simulink model "Segway"  (R2018b)
settings: Solver=VariableStepAuto  StartTime=0.0  StopTime=10.0  RelTol=1e-3
values from neighbouring files (symbols this model uses):
  a_1 = 1    [segway.m]
  beta0 = 2    [segway.m]
  l_p = 1    [segway.m]
  m_p = 1    [segway.m]
  m_w = 1.5    [segway.m]
  r = 0.2    [segway.m]
  theta0 = 0.6    [segway.m]
  theta_ref = 0.5    [segway.m]
undefined symbols (not defined in the file or in its folder): g, thetadot0
libraries: simulink x2
settings Model: Creator=Agurken  LastModifiedBy=Agurken
settings SolverCC: ZeroCrossAlgorithm=Adaptive
settings DebuggingCC: IgnoredZcDiagnostic=none

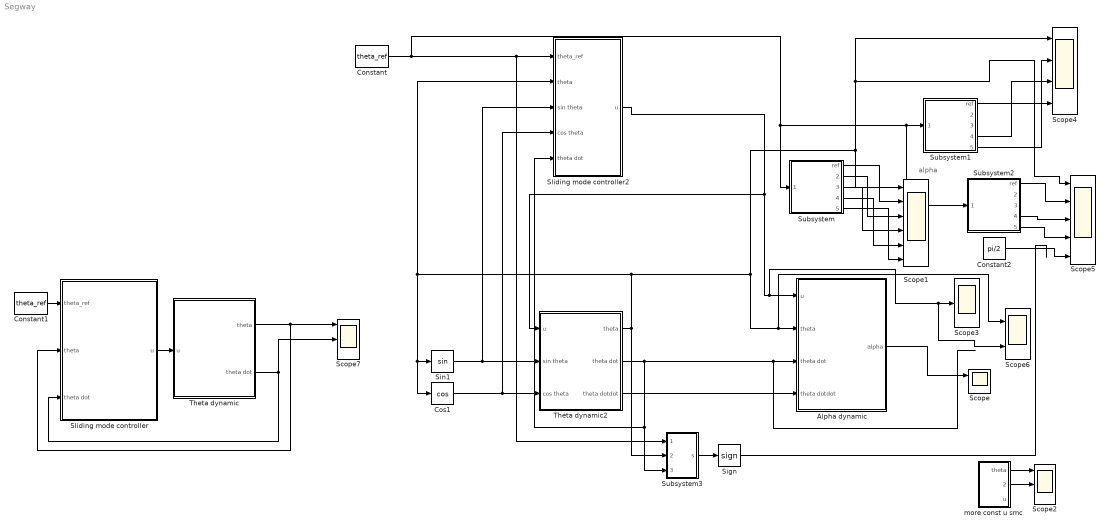
== system Segway ==
  note: alpha
  Alpha dynamic : Subsystem
  Constant : Constant  Value=theta_ref
  Constant1 : Constant  Value=theta_ref
  Constant2 : Constant  Value=pi/2
  Cos1 : Trigonometry  Operator=cos
  Scope : Scope  NumInputPorts=2
  Scope1 : Scope  NumInputPorts=6
  Scope2 : Scope  NumInputPorts=3
  Scope3 : Scope
  Scope4 : Scope  NumInputPorts=4
  Scope5 : Scope  NumInputPorts=5
  Scope6 : Scope  NumInputPorts=2
  Scope7 : Scope  NumInputPorts=3
  Sign : Signum
  Sin1 : Trigonometry
  Sliding mode controller : Subsystem
  Sliding mode controller2 : Subsystem
  Subsystem : Subsystem
  Subsystem1 : Subsystem
  Subsystem2 : Subsystem
  Subsystem3 : Subsystem
  Theta dynamic : Subsystem
  Theta dynamic2 : Subsystem
  more const u smc : Subsystem
  wires:
  Alpha dynamic/1(alpha) -> Scope/1
  Theta dynamic2/1("theta ") -> Subsystem3/2(theta), Sin1/1, Cos1/1, Sliding mode controller2/2(theta), Scope5/1, Scope4/1, Scope1/1, Scope6/1, Alpha dynamic/2(theta)
  Theta dynamic2/3("theta dotdot ") -> Alpha dynamic/4(theta dotdot)
  Cos1/1 -> Sliding mode controller2/4(cos theta), Theta dynamic2/3(cos theta)
  Sin1/1 -> Sliding mode controller2/3(sin theta), Theta dynamic2/2(sin theta)
  Sliding mode controller2/1(u) -> Scope6/2, Scope3/1, Alpha dynamic/1(u), Theta dynamic2/1(u)
  Constant/1 -> Subsystem3/1(theta_ref), Sliding mode controller2/1(theta_ref), Subsystem2/1(theta ref), Subsystem1/1(theta ref), Subsystem/1(theta ref)
  more const u smc/1(theta) -> Scope2/1
  more const u smc/2(theta ref) -> Scope2/2
  Subsystem/2(ref-eps) -> Scope1/3
  Subsystem/3(ref+epf) -> Scope1/4
  Subsystem/1(ref) -> Scope1/2
  Subsystem/5(ref+epf/a) -> Scope1/6
  Subsystem/4(ref-eps/a) -> Scope1/5
  Subsystem1/1(ref) -> Scope4/2
  Subsystem1/4(ref-eps/a) -> Scope4/3
  Subsystem1/5(ref+epf/a) -> Scope4/4
  Constant2/1 -> Scope5/5
  Subsystem2/4(ref-eps/a) -> Scope5/3
  Subsystem2/5(ref+epf/a) -> Scope5/4
  Subsystem2/1(ref) -> Scope5/2
  Subsystem3/1(s) -> Sign/1
  Sign/1 -> ?
  Sliding mode controller/1(u) -> Theta dynamic/1(u)
  Constant1/1 -> Sliding mode controller/1(theta_ref)
  Theta dynamic/1("theta ") -> Scope7/1, Sliding mode controller/2(theta)
  Theta dynamic/2("theta dot ") -> Scope7/2, Sliding mode controller/3(theta dot)
  Theta dynamic2/2("theta dot ") -> Subsystem3/3(theta dot), Sliding mode controller2/5(theta dot), Alpha dynamic/3(theta dot)

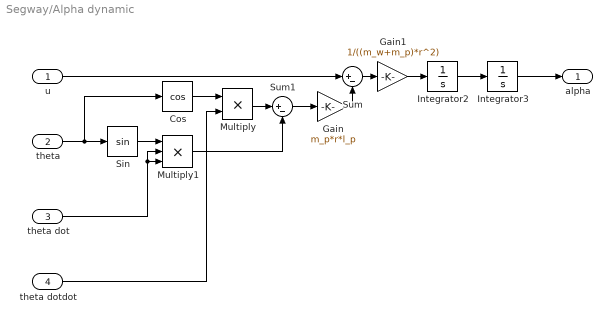
== system Segway/Alpha dynamic ==
  u : Inport
  theta : Inport  Port=2
  theta dot : Inport  Port=3
  theta dotdot : Inport  Port=4
  Cos : Trigonometry  Operator=cos
  Gain : Gain  Gain=m_p*r*l_p
  Gain1 : Gain  Gain=1/((m_w+m_p)*r^2)
  Integrator2 : Integrator
  Integrator3 : Integrator
  Multiply : Product
  Multiply1 : Product  Inputs=3
  Sin : Trigonometry
  Sum : Sum  Inputs=|+-
  Sum1 : Sum  Inputs=|+-
  alpha : Outport
  wires:
  Integrator2/1 -> Integrator3/1
  Multiply1/1 -> Sum1/2
  Multiply/1 -> Sum1/1
  Cos/1 -> Multiply/1
  Gain1/1 -> Integrator2/1
  Sin/1 -> Multiply1/1
  theta/1 -> Sin/1, Cos/1
  Sum1/1 -> Gain/1
  Sum/1 -> Gain1/1
  Gain/1 -> Sum/2
  u/1 -> Sum/1
  Integrator3/1 -> alpha/1
  theta dotdot/1 -> Multiply/2
  theta dot/1 -> Multiply1/3, Multiply1/2

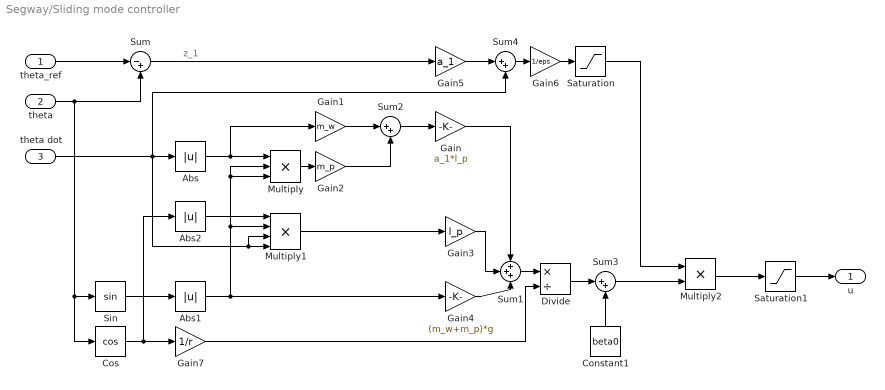
== system Segway/Sliding mode controller ==
  note: z_1
  theta_ref : Inport
  theta : Inport  Port=2
  theta dot : Inport  Port=3
  Abs : Abs
  Abs1 : Abs
  Abs2 : Abs
  Constant1 : Constant  Value=beta0
  Cos : Trigonometry  Operator=cos
  Divide : Product  Inputs=*/
  Gain : Gain  Gain=a_1*l_p
  Gain1 : Gain  Gain=m_w
  Gain2 : Gain  Gain=m_p
  Gain3 : Gain  Gain=l_p
  Gain4 : Gain  Gain=(m_w+m_p)*g
  Gain5 : Gain  Gain=a_1
  Gain6 : Gain  Gain=1/eps
  Gain7 : Gain  Gain=1/r
  Multiply : Product  Inputs=3
  Multiply1 : Product  Inputs=4
  Multiply2 : Product
  Saturation : Saturate  UpperLimit=1  LowerLimit=-1
  Saturation1 : Saturate  UpperLimit=1000  LowerLimit=-1000
  Sin : Trigonometry
  Sum : Sum  Inputs=|-+
  Sum1 : Sum  Inputs=3
  Sum2 : Sum  Inputs=|++
  Sum3 : Sum  Inputs=|++
  Sum4 : Sum  Inputs=|++
  u : Outport
  wires:
  Abs1/1 -> Multiply1/2, Multiply/3, Multiply/2, Gain4/1
  Sum1/1 -> Divide/1
  Sum2/1 -> Gain/1
  Sum3/1 -> Multiply2/2
  Gain3/1 -> Sum1/2
  theta dot/1 -> Multiply1/3, Multiply1/4, Abs/1, Sum4/2
  Gain6/1 -> Saturation/1
  Sum4/1 -> Gain6/1
  Multiply/1 -> Gain2/1
  Abs/1 -> Multiply/1, Gain1/1
  Saturation/1 -> Multiply2/1
  Gain2/1 -> Sum2/2
  Multiply2/1 -> Saturation1/1
  Multiply1/1 -> Gain3/1
  Gain5/1 -> Sum4/1
  Gain/1 -> Sum1/1
  Gain1/1 -> Sum2/1
  Gain4/1 -> Sum1/3
  Sin/1 -> Abs1/1
  Constant1/1 -> Sum3/2
  Cos/1 -> Gain7/1, Abs2/1
  theta/1 -> Cos/1, Sin/1, Sum/2
  theta_ref/1 -> Sum/1
  Gain7/1 -> Divide/2
  Divide/1 -> Sum3/1
  Saturation1/1 -> u/1
  Abs2/1 -> Multiply1/1
  Sum/1 -> Gain5/1

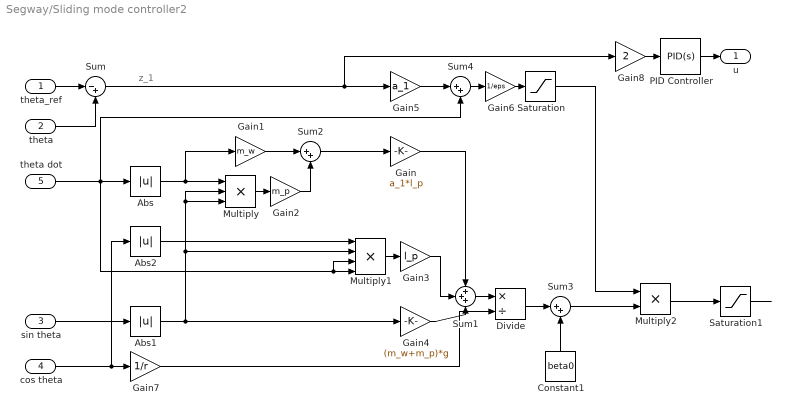
== system Segway/Sliding mode controller2 ==
  note: z_1
  theta_ref : Inport
  theta : Inport  Port=2
  sin theta : Inport  Port=3
  cos theta : Inport  Port=4
  theta dot : Inport  Port=5
  Abs : Abs
  Abs1 : Abs
  Abs2 : Abs
  Constant1 : Constant  Value=beta0
  Divide : Product  Inputs=*/
  Gain : Gain  Gain=a_1*l_p
  Gain1 : Gain  Gain=m_w
  Gain2 : Gain  Gain=m_p
  Gain3 : Gain  Gain=l_p
  Gain4 : Gain  Gain=(m_w+m_p)*g
  Gain5 : Gain  Gain=a_1
  Gain6 : Gain  Gain=1/eps
  Gain7 : Gain  Gain=1/r
  Gain8 : Gain  Gain=2
  Multiply : Product  Inputs=3
  Multiply1 : Product  Inputs=4
  Multiply2 : Product
  PID Controller : simulink/Continuous/PID Controller  Controller=PID  Form=Parallel  TimeDomain=Continuous-time  SampleTime=-1  IntegratorMethod=Forward Euler  FilterMethod=Forward Euler  ControllerParametersSource=internal  P=10  I=0  D=3  UseFilter=on  N=100  TunerSelectOption=Transfer Function Based (PID Tuner App)  InitialConditionSource=internal  InitialConditionForIntegrator=0  InitialConditionForFilter=0  DifferentiatorICPrevScaledInput=0  ExternalReset=none  TrackingMode=off  Kt=1  LimitOutput=off  UpperSaturationLimit=inf  LowerSaturationLimit=-inf  LinearizeAsGain=on  AntiWindupMode=none  Kb=1  POutMin=[]  POutMax=[]  IOutMin=[]  IOutMax=[]  DOutMin=[]  DOutMax=[]  NOutMin=[]  NOutMax=[]  SumOutMin=[]  SumOutMax=[]  SaturationOutMin=[]  SaturationOutMax=[]  PParamMin=[]  PParamMax=[]  IParamMin=[]  IParamMax=[]  DParamMin=[]  DParamMax=[]  NParamMin=[]  NParamMax=[]  KbParamMin=[]  KbParamMax=[]  KtParamMin=[]  KtParamMax=[]  KbOutMin=[]  KbOutMax=[]  KtOutMin=[]  KtOutMax=[]  IntegratorOutMin=[]  IntegratorOutMax=[]  FilterOutMin=[]  FilterOutMax=[]  SumI1OutMin=[]  SumI1OutMax=[]  SumI2OutMin=[]  SumI2OutMax=[]  SumI3OutMin=[]  SumI3OutMax=[]  SumI4OutMin=[]  SumI4OutMax=[]  SumDOutMin=[]  SumDOutMax=[]  DifferentiatorOutMin=[]  DifferentiatorOutMax=[]  FilterDiffOutCoefMin=[]  FilterDiffOutCoefMax=[]  ReciprocalOutMin=[]  ReciprocalOutMax=[]  SumDenOutMin=[]  SumDenOutMax=[]  SumNumOutMin=[]  SumNumOutMax=[]  DivideOutMin=[]  DivideOutMax=[]  IntegratorContinuousStateAttributes=''  IntegratorStateMustResolveToSignalObject=off  IntegratorRTWStateStorageClass=Auto  FilterContinuousStateAttributes=''  FilterStateMustResolveToSignalObject=off  FilterRTWStateStorageClass=Auto  ParallelPVariant=InternalParameters  IdealPVariant=Disabled  IVariant=InternalParameters  DVariant=InternalParameters  IntegratorVariant=Continuous  SatVariant=Disabled  AWVariant=Passthrough  PCopyVariant=Disabled  TRVariant=Disabled  FdbkBlocksVariant=Forward  IdealPFdbkVariant=Disabled  SatFdbkVariant=Disabled  DerivativeFilterVariant=ContFilter  NVariant=InternalParameters  NCopyVariant=Disabled  FilterICVariant=InternalICsFilter  IntegratorICVariant=InternalICs  ExternalResetVariant=Disabled  TRSumVariant=Passthrough  SumFdbkVariant=Disabled  SumVariant=Sum_PID
  Saturation : Saturate  UpperLimit=1  LowerLimit=-1
  Saturation1 : Saturate  UpperLimit=1000  LowerLimit=-1000
  Sum : Sum  Inputs=|-+
  Sum1 : Sum  Inputs=3
  Sum2 : Sum  Inputs=|++
  Sum3 : Sum  Inputs=|++
  Sum4 : Sum  Inputs=|++
  u : Outport
  wires:
  Abs1/1 -> Multiply1/2, Multiply/3, Multiply/2, Gain4/1
  Sum1/1 -> Divide/1
  Sum2/1 -> Gain/1
  Sum3/1 -> Multiply2/2
  Gain3/1 -> Sum1/2
  theta dot/1 -> Multiply1/4, Multiply1/3, Abs/1, Sum4/2
  Gain6/1 -> Saturation/1
  Sum4/1 -> Gain6/1
  Multiply/1 -> Gain2/1
  Abs/1 -> Multiply/1, Gain1/1
  Saturation/1 -> Multiply2/1
  Gain2/1 -> Sum2/2
  Multiply2/1 -> Saturation1/1
  Multiply1/1 -> Gain3/1
  Gain5/1 -> Sum4/1
  Gain/1 -> Sum1/1
  Gain1/1 -> Sum2/1
  Gain4/1 -> Sum1/3
  sin theta/1 -> Abs1/1
  Constant1/1 -> Sum3/2
  cos theta/1 -> Abs2/1, Gain7/1
  theta/1 -> Sum/2
  theta_ref/1 -> Sum/1
  Divide/1 -> Sum3/1
  Saturation1/1 -> ?
  Abs2/1 -> Multiply1/1
  PID Controller/1 -> u/1
  Sum/1 -> Gain8/1, Gain5/1
  Gain7/1 -> Divide/2
  Gain8/1 -> PID Controller/1

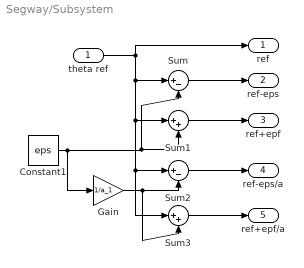
== system Segway/Subsystem ==
  theta ref : Inport
  Constant1 : Constant  Value=eps
  Gain : Gain  Gain=1/a_1
  Sum : Sum  Inputs=|+-
  Sum1 : Sum  Inputs=|++
  Sum2 : Sum  Inputs=|+-
  Sum3 : Sum  Inputs=|++
  ref : Outport
  ref-eps : Outport  Port=2
  ref+epf : Outport  Port=3
  ref-eps/a : Outport  Port=4
  ref+epf/a : Outport  Port=5
  wires:
  Sum1/1 -> ref+epf/1
  Constant1/1 -> Gain/1, Sum/2, Sum1/2
  Sum/1 -> ref-eps/1
  theta ref/1 -> ref/1, Sum/1, Sum1/1, Sum2/1, Sum3/1
  Gain/1 -> Sum3/2, Sum2/2
  Sum2/1 -> ref-eps/a/1
  Sum3/1 -> ref+epf/a/1

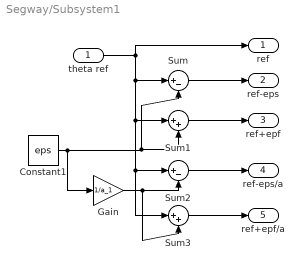
== system Segway/Subsystem1 ==
  theta ref : Inport
  Constant1 : Constant  Value=eps
  Gain : Gain  Gain=1/a_1
  Sum : Sum  Inputs=|+-
  Sum1 : Sum  Inputs=|++
  Sum2 : Sum  Inputs=|+-
  Sum3 : Sum  Inputs=|++
  ref : Outport
  ref-eps : Outport  Port=2
  ref+epf : Outport  Port=3
  ref-eps/a : Outport  Port=4
  ref+epf/a : Outport  Port=5
  wires:
  Sum1/1 -> ref+epf/1
  Constant1/1 -> Gain/1, Sum/2, Sum1/2
  Sum/1 -> ref-eps/1
  theta ref/1 -> ref/1, Sum/1, Sum1/1, Sum2/1, Sum3/1
  Gain/1 -> Sum3/2, Sum2/2
  Sum2/1 -> ref-eps/a/1
  Sum3/1 -> ref+epf/a/1

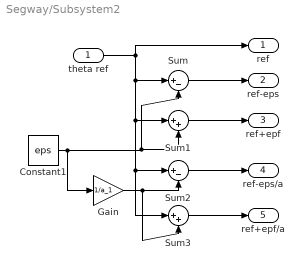
== system Segway/Subsystem2 ==
  theta ref : Inport
  Constant1 : Constant  Value=eps
  Gain : Gain  Gain=1/a_1
  Sum : Sum  Inputs=|+-
  Sum1 : Sum  Inputs=|++
  Sum2 : Sum  Inputs=|+-
  Sum3 : Sum  Inputs=|++
  ref : Outport
  ref-eps : Outport  Port=2
  ref+epf : Outport  Port=3
  ref-eps/a : Outport  Port=4
  ref+epf/a : Outport  Port=5
  wires:
  Sum1/1 -> ref+epf/1
  Constant1/1 -> Gain/1, Sum/2, Sum1/2
  Sum/1 -> ref-eps/1
  theta ref/1 -> ref/1, Sum/1, Sum1/1, Sum2/1, Sum3/1
  Gain/1 -> Sum3/2, Sum2/2
  Sum2/1 -> ref-eps/a/1
  Sum3/1 -> ref+epf/a/1

== system Segway/Subsystem3 ==
  theta_ref : Inport
  theta : Inport  Port=2
  theta dot : Inport  Port=3
  Gain : Gain  Gain=a_1
  Sum : Sum  Inputs=|+-
  Sum1 : Sum  Inputs=|++
  s : Outport
  wires:
  Sum/1 -> Gain/1
  Gain/1 -> Sum1/2
  theta_ref/1 -> Sum/2
  Sum1/1 -> s/1
  theta dot/1 -> Sum1/1
  theta/1 -> Sum/1

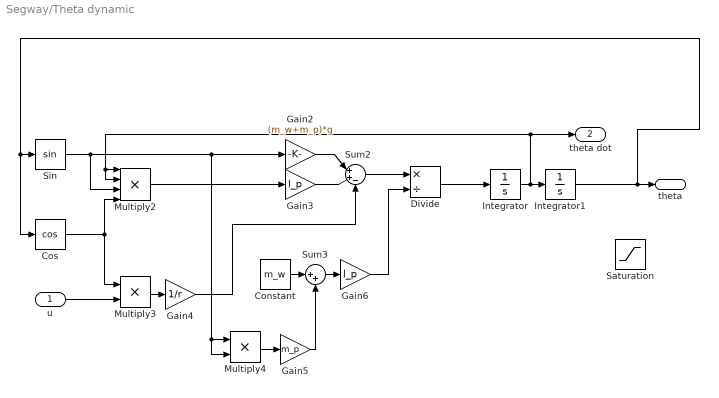
== system Segway/Theta dynamic ==
  u : Inport
  Constant : Constant  Value=m_w
  Cos : Trigonometry  Operator=cos
  Divide : Product  Inputs=*/
  Gain2 : Gain  Gain=(m_w+m_p)*g
  Gain3 : Gain  Gain=l_p
  Gain4 : Gain  Gain=1/r
  Gain5 : Gain  Gain=m_p
  Gain6 : Gain  Gain=l_p
  Integrator : Integrator  InitialCondition=thetadot0
  Integrator1 : Integrator  InitialCondition=theta0
  Multiply2 : Product  Inputs=4
  Multiply3 : Product
  Multiply4 : Product
  Saturation : Saturate  UpperLimit=pi-eps  LowerLimit=-pi+eps
  Sin : Trigonometry
  Sum2 : Sum  Inputs=|++-
  Sum3 : Sum  Inputs=|++
  "theta " : Outport
  "theta dot " : Outport  Port=2
  wires:
  Sum3/1 -> Gain6/1
  Sin/1 -> Gain2/1, Multiply4/1, Multiply4/2, Multiply2/3
  Divide/1 -> Integrator/1
  Multiply2/1 -> Gain3/1
  Gain3/1 -> Sum2/2
  Integrator/1 -> "theta dot "/1, Multiply2/2, Multiply2/1, Integrator1/1
  Gain2/1 -> Sum2/1
  Cos/1 -> Multiply3/1, Multiply2/4
  Gain5/1 -> Sum3/2
  Multiply3/1 -> Gain4/1
  Multiply4/1 -> Gain5/1
  Constant/1 -> Sum3/1
  Sum2/1 -> Divide/1
  u/1 -> Multiply3/2
  Gain4/1 -> Sum2/3
  Gain6/1 -> Divide/2
  Integrator1/1 -> Cos/1, Sin/1, "theta "/1

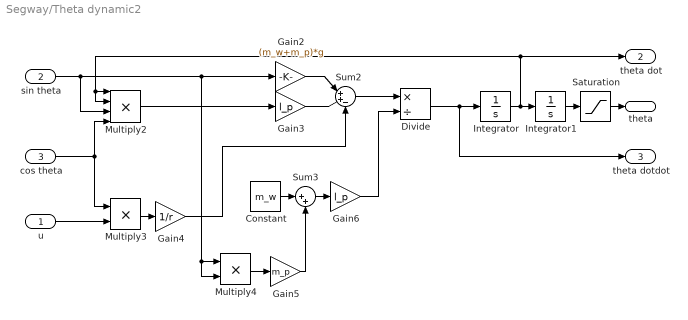
== system Segway/Theta dynamic2 ==
  u : Inport
  sin theta : Inport  Port=2
  cos theta : Inport  Port=3
  Constant : Constant  Value=m_w
  Divide : Product  Inputs=*/
  Gain2 : Gain  Gain=(m_w+m_p)*g
  Gain3 : Gain  Gain=l_p
  Gain4 : Gain  Gain=1/r
  Gain5 : Gain  Gain=m_p
  Gain6 : Gain  Gain=l_p
  Integrator : Integrator
  Integrator1 : Integrator  InitialCondition=theta0
  Multiply2 : Product  Inputs=4
  Multiply3 : Product
  Multiply4 : Product
  Saturation : Saturate  UpperLimit=pi-eps  LowerLimit=-pi+eps
  Sum2 : Sum  Inputs=|++-
  Sum3 : Sum  Inputs=|++
  "theta " : Outport
  "theta dot " : Outport  Port=2
  "theta dotdot " : Outport  Port=3
  wires:
  Sum3/1 -> Gain6/1
  sin theta/1 -> Gain2/1, Multiply4/1, Multiply4/2, Multiply2/3
  Divide/1 -> "theta dotdot "/1, Integrator/1
  Multiply2/1 -> Gain3/1
  Gain3/1 -> Sum2/2
  Integrator/1 -> "theta dot "/1, Multiply2/2, Multiply2/1, Integrator1/1
  Gain2/1 -> Sum2/1
  Integrator1/1 -> Saturation/1
  cos theta/1 -> Multiply3/1, Multiply2/4
  Gain5/1 -> Sum3/2
  Multiply3/1 -> Gain4/1
  Multiply4/1 -> Gain5/1
  Constant/1 -> Sum3/1
  Sum2/1 -> Divide/1
  u/1 -> Multiply3/2
  Gain4/1 -> Sum2/3
  Gain6/1 -> Divide/2
  Saturation/1 -> "theta "/1

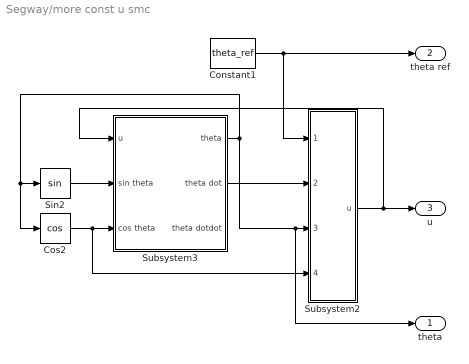
== system Segway/more const u smc ==
  Constant1 : Constant  Value=theta_ref
  Cos2 : Trigonometry  Operator=cos
  Sin2 : Trigonometry
  Subsystem2 : Subsystem
  Subsystem3 : Subsystem
  theta : Outport
  theta ref : Outport  Port=2
  u : Outport  Port=3
  wires:
  Sin2/1 -> Subsystem3/2(sin theta)
  Cos2/1 -> Subsystem2/4(cos theta), Subsystem3/3(cos theta)
  Subsystem2/1(u) -> u/1, Subsystem3/1(u)
  Subsystem3/1("theta ") -> Sin2/1, Cos2/1, theta/1, Subsystem2/3(theta)
  Constant1/1 -> Subsystem2/1(theta_ref), theta ref/1
  Subsystem3/2("theta dot ") -> Subsystem2/2(theta dot)

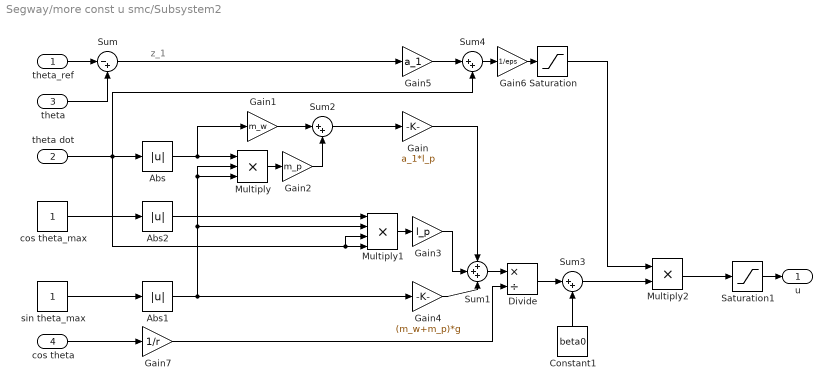
== system Segway/more const u smc/Subsystem2 ==
  note: z_1
  theta_ref : Inport
  theta dot : Inport  Port=2
  theta : Inport  Port=3
  cos theta : Inport  Port=4
  Abs : Abs
  Abs1 : Abs
  Abs2 : Abs
  Constant1 : Constant  Value=beta0
  Divide : Product  Inputs=*/
  Gain : Gain  Gain=a_1*l_p
  Gain1 : Gain  Gain=m_w
  Gain2 : Gain  Gain=m_p
  Gain3 : Gain  Gain=l_p
  Gain4 : Gain  Gain=(m_w+m_p)*g
  Gain5 : Gain  Gain=a_1
  Gain6 : Gain  Gain=1/eps
  Gain7 : Gain  Gain=1/r
  Multiply : Product  Inputs=3
  Multiply1 : Product  Inputs=4
  Multiply2 : Product
  Saturation : Saturate  UpperLimit=1  LowerLimit=-1
  Saturation1 : Saturate  UpperLimit=1000  LowerLimit=-1000
  Sum : Sum  Inputs=|-+
  Sum1 : Sum  Inputs=3
  Sum2 : Sum  Inputs=|++
  Sum3 : Sum  Inputs=|++
  Sum4 : Sum  Inputs=|++
  cos theta_max : Constant
  sin theta_max : Constant
  u : Outport
  wires:
  Abs1/1 -> Multiply1/2, Multiply/3, Multiply/2, Gain4/1
  Sum1/1 -> Divide/1
  Sum2/1 -> Gain/1
  Sum3/1 -> Multiply2/2
  Sum/1 -> Gain5/1
  Gain3/1 -> Sum1/2
  theta dot/1 -> Multiply1/4, Multiply1/3, Abs/1, Sum4/2
  Gain6/1 -> Saturation/1
  Sum4/1 -> Gain6/1
  Multiply/1 -> Gain2/1
  Abs/1 -> Multiply/1, Gain1/1
  Saturation/1 -> Multiply2/1
  Gain2/1 -> Sum2/2
  Multiply2/1 -> Saturation1/1
  Multiply1/1 -> Gain3/1
  Gain5/1 -> Sum4/1
  Gain/1 -> Sum1/1
  Gain1/1 -> Sum2/1
  Gain4/1 -> Sum1/3
  sin theta_max/1 -> Abs1/1
  Constant1/1 -> Sum3/2
  cos theta/1 -> Gain7/1
  theta/1 -> Sum/2
  theta_ref/1 -> Sum/1
  Gain7/1 -> Divide/2
  Divide/1 -> Sum3/1
  Saturation1/1 -> u/1
  Abs2/1 -> Multiply1/1
  cos theta_max/1 -> Abs2/1

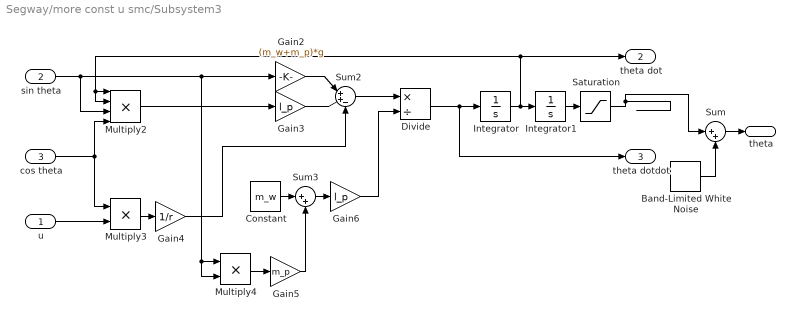
== system Segway/more const u smc/Subsystem3 ==
  u : Inport
  sin theta : Inport  Port=2
  cos theta : Inport  Port=3
  Band-Limited White Noise : simulink/Sources/Band-Limited White Noise  Cov=[0.1]  Ts=0.1  seed=[23341]
  Constant : Constant  Value=m_w
  Divide : Product  Inputs=*/
  Gain2 : Gain  Gain=(m_w+m_p)*g
  Gain3 : Gain  Gain=l_p
  Gain4 : Gain  Gain=1/r
  Gain5 : Gain  Gain=m_p
  Gain6 : Gain  Gain=l_p
  Integrator : Integrator
  Integrator1 : Integrator  InitialCondition=theta0
  Multiply2 : Product  Inputs=4
  Multiply3 : Product
  Multiply4 : Product
  Saturation : Saturate  UpperLimit=pi-eps  LowerLimit=-pi+eps
  Sum : Sum  Inputs=|++
  Sum2 : Sum  Inputs=|++-
  Sum3 : Sum  Inputs=|++
  "theta " : Outport
  "theta dot " : Outport  Port=2
  "theta dotdot " : Outport  Port=3
  wires:
  Sum3/1 -> Gain6/1
  sin theta/1 -> Gain2/1, Multiply4/1, Multiply4/2, Multiply2/3
  Divide/1 -> "theta dotdot "/1, Integrator/1
  Multiply2/1 -> Gain3/1
  Gain3/1 -> Sum2/2
  Integrator/1 -> "theta dot "/1, Multiply2/2, Multiply2/1, Integrator1/1
  Gain2/1 -> Sum2/1
  Integrator1/1 -> Saturation/1
  cos theta/1 -> Multiply3/1, Multiply2/4
  Gain5/1 -> Sum3/2
  Multiply3/1 -> Gain4/1
  Multiply4/1 -> Gain5/1
  Constant/1 -> Sum3/1
  Sum2/1 -> Divide/1
  u/1 -> Multiply3/2
  Gain4/1 -> Sum2/3
  Gain6/1 -> Divide/2
  Saturation/1 -> Sum/1
  Band-Limited White Noise/1 -> Sum/2
  Sum/1 -> "theta "/1
